simulink model "Problem9"  (R2020b)
settings: Solver=VariableStepAuto  StartTime=0.0  StopTime=10.0  RelTol=1e-3
undefined symbols (not defined in the file): Ke, Kt
settings Model: Creator=sonal  LastModifiedBy=sonal

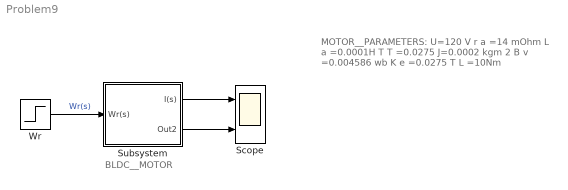
== system Problem9 ==
  note: MOTOR__PARAMETERS:
      | U=120 V
      | r a =14 mOhm
      | L a =0.0001H
      | T T =0.0275
      | J=0.0002 kgm 2
      | B v =0.004586 wb
      | K e =0.0275
      | T L =10Nm
  note: BLDC__MOTOR
  Scope : Scope  NumInputPorts=2
  Subsystem : Subsystem
  Wr : Step  SampleTime=0
  wires:
  Subsystem/2(Out2) -> Scope/2
  Wr/1 -> Subsystem/1(Wr(s))  "Wr(s)"
  Subsystem/1(I(s)) -> Scope/1

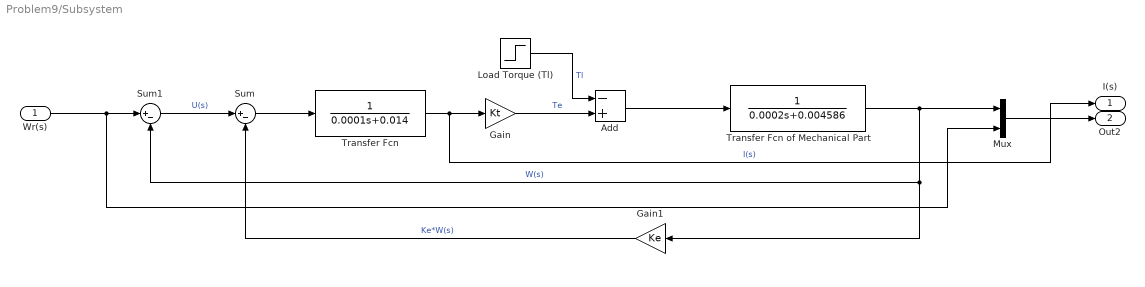
== system Problem9/Subsystem ==
  Wr(s) : Inport
  Add : Sum  Inputs=-+
  Gain : Gain  Gain=Kt
  Gain1 : Gain  Gain=Ke
  Load Torque (Tl) : Step  SampleTime=0
  Mux : Mux  Inputs=2
  Sum : Sum  Inputs=|+-
  Sum1 : Sum  Inputs=|+-
  "Transfer Fcn " : TransferFcn  Denominator=[0.0001 0.014]
  Transfer Fcn of Mechanical Part : TransferFcn  Denominator=[0.0002 0.004586]
  I(s) : Outport
  Out2 : Outport  Port=2
  wires:
  Mux/1 -> Out2/1
  Load Torque (Tl)/1 -> Add/1  "Tl"
  Sum/1 -> "Transfer Fcn "/1
  Wr(s)/1 -> Mux/2, Sum1/1
  "Transfer Fcn "/1 -> I(s)/1, Gain/1  "I(s)"
  Transfer Fcn of Mechanical Part/1 -> Mux/1, Gain1/1, Sum1/2  "W(s)"
  Add/1 -> Transfer Fcn of Mechanical Part/1
  Gain/1 -> Add/2  "Te"
  Gain1/1 -> Sum/2  "Ke*W(s)"
  Sum1/1 -> Sum/1  "U(s)"
